simulink model "clarke"  (R2023b)
settings: Solver=VariableStepAuto  StartTime=0.0  StopTime=10.0  RelTol=1e-3
libraries: mcbcontrolslib x2
settings Model: Creator=JUEMING  LastModifiedBy=JUEMING_SHI
settings SolverCC: AlgebraicLoopSolver=TrustRegion
settings DataIOCC: ReturnWorkspaceOutputs=off
settings DebuggingCC: UnconnectedInputMsg=warning  UnconnectedOutputMsg=warning  UnconnectedLineMsg=warning  ArithmeticOperatorsInVariantConditions=warning
settings ModelReferenceCC: EnableRefExpFcnMdlSchedulingChecks=on
settings SFSimCC: CustomCodeUndefinedFunction=UseInterfaceOnly

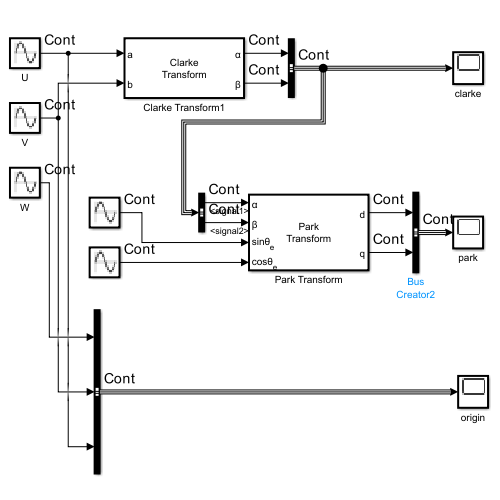
[thumbnail: Simulink's stored preview of the top-level diagram]
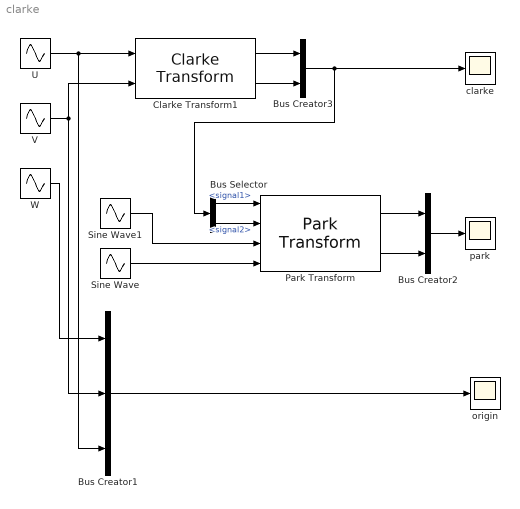
== system clarke ==
  Bus Creator1 : BusCreator  Inputs=3
  Bus Creator2 : BusCreator  Inputs=2
  Bus Creator3 : BusCreator  Inputs=2
  Bus Selector : BusSelector  OutputSignals=signal1,signal2
  Clarke Transform1 : mcbcontrolslib/Clarke Transform  VariantControl=Variant2  PhaseInput=Two inputs  EnPowerInv=off
      settings: LibrarySourceBlock=mcblib/Controls/Math Transforms/Clarke Transform
  Park Transform : mcbcontrolslib/Park Transform  PhaseInput=Two inputs  AxisAlignment=D-axis  ThetaInput=Sine and Cosine electrical position  AngleInput=Per-unit  N_points=1024
      settings: LibrarySourceBlock=mcblib/Controls/Math Transforms/Park Transform
  Sine Wave : Sin  Phase=pi/2  SampleTime=0
  Sine Wave1 : Sin  SampleTime=0
  U : Sin  SampleTime=0
  V : Sin  Phase=pi*2/3  SampleTime=0
  W : Sin  Phase=pi*4/3  SampleTime=0
  clarke : Scope
  origin : Scope
  park : Scope
  wires:
  V/1 -> Clarke Transform1/2, Bus Creator1/2
  W/1 -> Bus Creator1/1
  Bus Creator1/1 -> origin/1
  Park Transform/2 -> Bus Creator2/2
  Park Transform/1 -> Bus Creator2/1
  Bus Creator2/1 -> park/1
  Bus Selector/1 -> Park Transform/1  "<signal1>"
  Bus Selector/2 -> Park Transform/2  "<signal2>"
  Sine Wave1/1 -> Park Transform/3
  Sine Wave/1 -> Park Transform/4
  U/1 -> Clarke Transform1/1, Bus Creator1/3
  Clarke Transform1/2 -> Bus Creator3/2
  Clarke Transform1/1 -> Bus Creator3/1
  Bus Creator3/1 -> Bus Selector/1, clarke/1
